simulink model "Function_Code"  (R2022a)
settings: Solver=VariableStepAuto  StartTime=0.0  StopTime=10.0  RelTol=1e-3
libraries: arduinolib x1
settings Model: Creator=19189  LastModifiedBy=19189

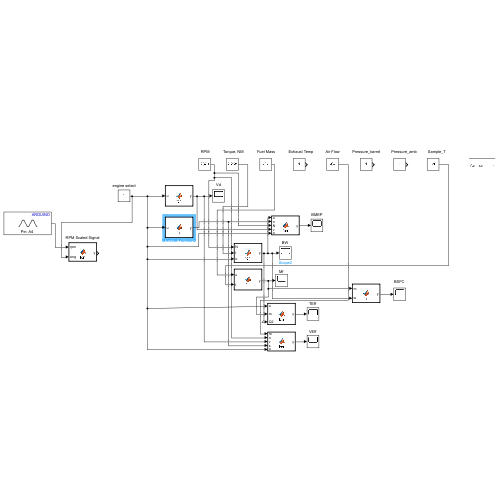
[thumbnail: Simulink's stored preview of the top-level diagram]
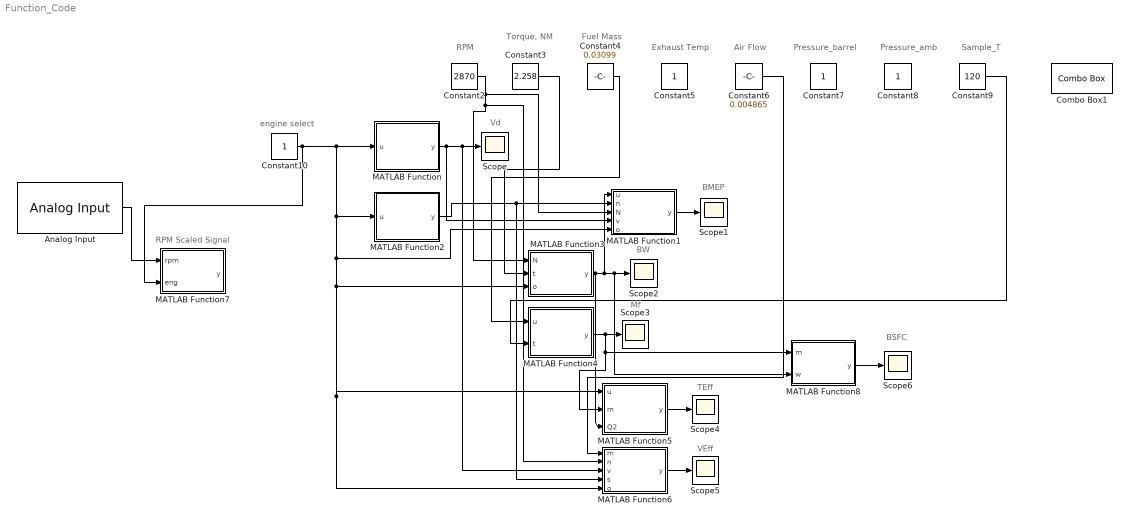
== system Function_Code ==
  note: BSFC
  note: RPM Scaled Signal
  note: engine select
  note: VEff
  note: TEff
  note: Mf
  note: Sample_T
  note: BW
  note: BMEP
  note: Vd
  note: Pressure_amb
  note: Pressure_barrel
  note: Air Flow
  note: Exhaust Temp
  note: Fuel Mass
  note: Torque, NM
  note: RPM
  Analog Input : arduinolib/Analog Input  pinNumber=4  ReadResultsOnly=off  ConversionTriggerSource=Software  ExternalTriggerType=uint32( 0 )  OutputDataType=uint16  EnableConversionCompleteNotify=off  EnableOuputStatus=off  SampleTime=-1  blockPlatform=arduino
  Combo Box1 : ComboBox  LabelPosition=Hide  SelectedLabel=Yanmar
      settings: Values={{'Yanmar', 'Craftsman', 'John Deer', 'Chevy V6', 'Kohler', 'DuroMax'}, [1 2 3 4 5 6]}
  Constant{5,7..8,10} (4 alike) : Constant
  Constant2 : Constant  Value=2870
  Constant3 : Constant  Value=2.258
  Constant4 : Constant  Value=0.03099
  Constant6 : Constant  Value=0.004865
  Constant9 : Constant  Value=120
  MATLAB Function : MATLAB Function  TreatAsAtomicUnit=on
  MATLAB Function1 : MATLAB Function  TreatAsAtomicUnit=on
  MATLAB Function2 : MATLAB Function  TreatAsAtomicUnit=on
  MATLAB Function3 : MATLAB Function  TreatAsAtomicUnit=on
  MATLAB Function4 : MATLAB Function  TreatAsAtomicUnit=on
  MATLAB Function5 : MATLAB Function  TreatAsAtomicUnit=on
  MATLAB Function6 : MATLAB Function  TreatAsAtomicUnit=on
  MATLAB Function7 : MATLAB Function  TreatAsAtomicUnit=on
  MATLAB Function8 : MATLAB Function  TreatAsAtomicUnit=on
  Scope{,1..6} (7 alike) : Scope
  wires:
  MATLAB Function/1(y) -> MATLAB Function1/4(v), MATLAB Function6/3(v), Scope/1
  Constant10/1 -> MATLAB Function7/2(eng), MATLAB Function1/5(o), MATLAB Function3/3(o), MATLAB Function6/5(o), MATLAB Function5/1(u), MATLAB Function2/1(u), MATLAB Function/1(u)
  Constant3/1 -> MATLAB Function3/2(t)
  MATLAB Function2/1(y) -> MATLAB Function6/4(s), MATLAB Function1/2(n)
  MATLAB Function1/1(y) -> Scope1/1
  Constant2/1 -> MATLAB Function1/3(N), MATLAB Function6/2(n), MATLAB Function3/1(N)
  MATLAB Function3/1(y) -> MATLAB Function5/3(Q2), MATLAB Function1/1(u), MATLAB Function8/2(w), Scope2/1
  Constant4/1 -> MATLAB Function4/1(u)
  Constant9/1 -> MATLAB Function4/2(t)
  MATLAB Function4/1(y) -> MATLAB Function5/2(m), MATLAB Function8/1(m), Scope3/1
  MATLAB Function5/1(y) -> Scope4/1
  Constant6/1 -> MATLAB Function6/1(m)
  MATLAB Function6/1(y) -> Scope5/1
  Analog Input/1 -> MATLAB Function7/1(rpm)
  MATLAB Function8/1(y) -> Scope6/1

== matlab function Function_Code/MATLAB Function1 ==
  data: u input; y output; n input; N input; v input; o input
function y = fcn(u, n, N,  v, o)
if(o == 1 || o == 2 || o == 5 || o ==6)
    y = ((u/((N/60)/n))/v)/1000;
elseif(o==3)
     y = ((u/((N/60)/n))/(v*4))/1000;
else
     y = ((u/((N/60)/n))/(v*6))/1000;
end

== matlab function Function_Code/MATLAB Function ==
  data: y output; u input
function y = fcn(u)
data = [0.000296 0.000196 0.000475 000.0004667 0.000429 0.000225];

y = data(1,u);

== matlab function Function_Code/MATLAB Function2 ==
  data: y output; u input
function y = fcn(u)
data = [4  4  4  4 4 4];

y = data(1,u);

== matlab function Function_Code/MATLAB Function3 ==
  data: N input; y output; t input; o input
function y = fcn(N,t, o)
if(o == 1 ||  o == 2 || o == 5 || o ==6)
    y = 2 * pi * (N/60.0) * t;

elseif(o == 3)
    y = 2 * pi * (N/60.0) * t * 4;
else
    y = 2 * pi * (N/60.0) * t * 6;
end

== matlab function Function_Code/MATLAB Function4 ==
  data: y output; u input; t input
function y = fcn(u, t)

y = u/(t);

== matlab function Function_Code/MATLAB Function5 ==
  data: y output; u input; m input; Q2 input
function y = fcn(u, m, Q2)
data = [47.3e6 44.4e6];
Q1 = 0;
if(u == 3)
    Q1 = m * data(1, 2);

else
    Q1 = m * data(1,1);
end

y = (Q2/Q1) * 100;

== matlab function Function_Code/MATLAB Function6 ==
  data: m input; y output; n input; v input; s input; o input
function y = fcn(m, n, v, s,o)
if(o == 1 || o == 2 || o == 5 || o == 6)
    y = ((s*m)/(1.205*v*(n/60)));
elseif (o == 3)
    y = ((s*m)/(1.205*(v*4)*(n/60)));
else
    y = ((s*m)/(1.205*(v*6)*(n/60)));
end

== matlab function Function_Code/MATLAB Function7 ==
  data: rpm input; y output; eng input
function y = fcn(rpm,eng)

if(eng ==1)
   y = (rpm/1023.0)*(2839-2937.5) + 2937.5;
elseif(eng == 2)
    y = (rpm/1023.0)*(3499.1-3752.7) + 3752.7;
elseif(eng == 3)
    y = (rpm/1023.0)*(1); %%fix me
elseif(eng == 4)
    y = (rpm/1023.0)*(858-398.3) + 398.3;
else
    y = 0;
end

== matlab function Function_Code/MATLAB Function8 ==
  data: m input; y output; w input
function y = fcn(m,w)

y = u;
